simulink model "Hauteur_Capteurs"  (R2021a)
settings: Solver=FixedStepAuto  StartTime=0.0  StopTime=10.0  RelTol=1e-3
values from neighbouring files (symbols this model uses):
  Xd = r_def*sind(30)    [Hauteur_Aimants_Plaque.m]    (also in Hauteur_Aimants_Plaque_calculs.m = r_def*sin(deg2rad(30)))
  Xe = -r_def*sind(30)    [Hauteur_Aimants_Plaque.m]    (also in Hauteur_Aimants_Plaque_calculs.m = -0.08)
  Xf = r_def*sind(30)    [Hauteur_Aimants_Plaque.m]    (also in Hauteur_Aimants_Plaque_calculs.m = r_def*sin(deg2rad(30)))
  Yd = r_def*cosd(30)    [Hauteur_Aimants_Plaque.m]    (also in Hauteur_Aimants_Plaque_calculs.m = r_def*cos(deg2rad(30)))
  Ye = 0    [Hauteur_Aimants_Plaque.m]    (also in Hauteur_Aimants_Plaque_calculs.m)
  Yf = -r_def*cosd(30)    [Hauteur_Aimants_Plaque.m]    (also in Hauteur_Aimants_Plaque_calculs.m = -r_def*cos(deg2rad(30)))
settings Model: Creator=antho  LastModifiedBy=antho

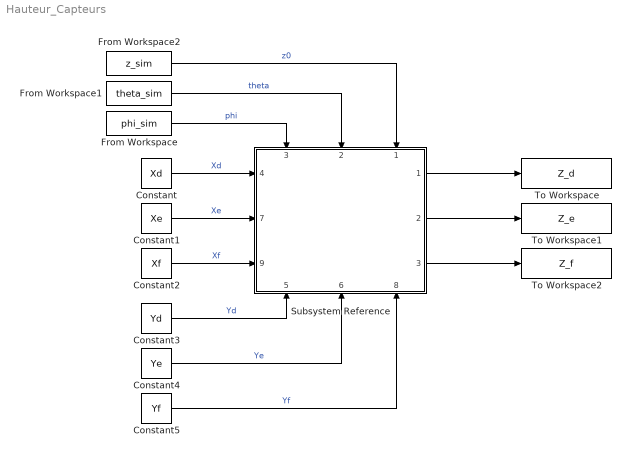
== system Hauteur_Capteurs ==
  Constant : Constant  Value=Xd
  Constant1 : Constant  Value=Xe
  Constant2 : Constant  Value=Xf
  Constant3 : Constant  Value=Yd
  Constant4 : Constant  Value=Ye
  Constant5 : Constant  Value=Yf
  From Workspace : FromWorkspace  VariableName=phi_sim
  From Workspace1 : FromWorkspace  VariableName=theta_sim
  From Workspace2 : FromWorkspace  VariableName=z_sim
  Subsystem Reference : Subsystem  ReferencedSubsystem=subsys_calcul_capteurs
      settings: PortSchema="{\"entries\":[{\"content\":{\"sides\":[{\"content\":{\"connectorIds\":[\"In4\",\"In7\",\"In9\"]},\"type\":\"ConnectorPlacement.EquallySpacedRectSide\",\"uuid\":\"7742b6ab-e25f-4596-812b-32c482f36de2\"},{\"content\":{\"connectorIds\":[\"Out1\",\"Out2\",\"Out3\"],\"side\":\"RIGHT\"},\"type\":\"ConnectorPlacement.EquallySpacedRectSide\",\"uuid\":\"e42faa24-2954-4ddc-a361-b06612dcf128\"},{\"content\":{\"connectorIds\":[\"In3\",\"In2\",\"In1\"],\"side\":\"TOP\"},\"type\":\"ConnectorPlacement.EquallySpacedRectSide\",\"uuid\":\"b7ccb92e-d184-4db5-9be8-b7d4d28bfe4b\"},{\"content\":{\"connectorIds\":[\"In5\",\"In6\",\"In8\"],\"side\":\"BOTTOM\"},\"type\":\"ConnectorPlacement.EquallySpacedRectSide\",\"uuid\":\"3e09f896-ea69-4de4-a00a-62031f57fff3\"}]},\"type\":\"ConnectorPlacement.EquallySpacedConnector\",\"uuid\":\"f30a8a90-6e1f-48e7-abc9-dd24ec852e72\"}],\"packageUris\":[\"http://schema.mathworks.com/mf0/Connector/R2020b\"],\"version\":\"1.0\"}"
  To Workspace : ToWorkspace  VariableName=Z_d  SaveFormat=Timeseries  SampleTime=-1
  To Workspace1 : ToWorkspace  VariableName=Z_e  SaveFormat=Timeseries  SampleTime=-1
  To Workspace2 : ToWorkspace  VariableName=Z_f  SaveFormat=Timeseries  SampleTime=-1
  wires:
  From Workspace2/1 -> Subsystem Reference/1  "z0"
  From Workspace1/1 -> Subsystem Reference/2  "theta"
  From Workspace/1 -> Subsystem Reference/3  "phi"
  Subsystem Reference/1 -> To Workspace/1
  Subsystem Reference/2 -> To Workspace1/1
  Subsystem Reference/3 -> To Workspace2/1
  Constant2/1 -> Subsystem Reference/9  "Xf"
  Constant1/1 -> Subsystem Reference/7  "Xe"
  Constant/1 -> Subsystem Reference/4  "Xd"
  Constant3/1 -> Subsystem Reference/5  "Yd"
  Constant5/1 -> Subsystem Reference/8  "Yf"
  Constant4/1 -> Subsystem Reference/6  "Ye"
